simulink model "Example1_sim_"  (R2019b)
settings: Solver=ode4  StartTime=0.0  StopTime=10.0  FixedStep=0.001  RelTol=1e-3
values from neighbouring files (symbols this model uses):
  A = [0 2;0 3]    [Example1_.m]
  B = [0;1]    [Example1_.m]
  K = acker(A,B,desired_poles)    [Example1_.m]
settings Model: Creator=Aria  LastModifiedBy=Aria

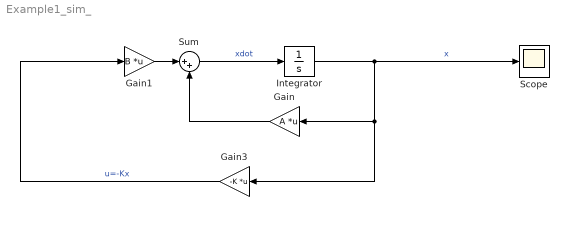
== system Example1_sim_ ==
  Gain : Gain  Gain=A  Multiplication=Matrix(K*u)
  Gain1 : Gain  Gain=B  Multiplication=Matrix(K*u)
  Gain3 : Gain  Gain=-K  Multiplication=Matrix(K*u)
  Integrator : Integrator  InitialCondition=[1;5]
  Scope : Scope
  Sum : Sum  Inputs=|++
  wires:
  Sum/1 -> Integrator/1  "xdot"
  Gain/1 -> Sum/2
  Gain3/1 -> Gain1/1  "u=-Kx"
  Gain1/1 -> Sum/1
  Integrator/1 -> Scope/1, Gain3/1, Gain/1  "x"
